simulink subsystem "invertedPendulum"  (R2024a)
settings: Solver=VariableStepAuto  StartTime=0.0  StopTime=10.0  RelTol=1e-3
undefined symbols (not defined in the file): I, L, m, M
settings Model: Creator=Peter  LastModifiedBy=Peter

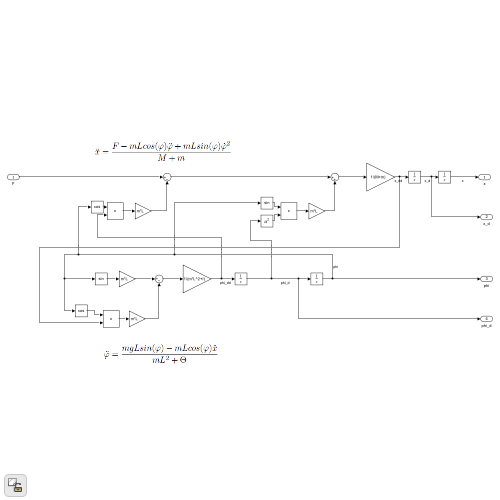
[thumbnail: Simulink's stored preview of the top-level diagram]
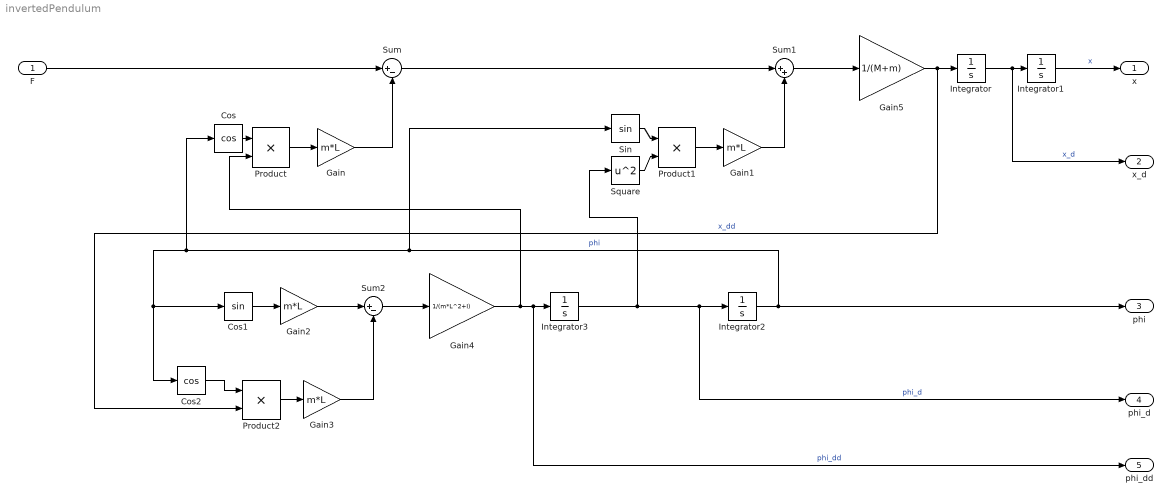
== system invertedPendulum ==
  F : Inport
  Cos : Trigonometry  Operator=cos
  Cos1 : Trigonometry
  Cos2 : Trigonometry  Operator=cos
  Gain{,1..3} (4 alike) : Gain  Gain=m*L
  Gain4 : Gain  Gain=1/(m*L^2+I)
  Gain5 : Gain  Gain=1/(M+m)
  Integrator{,1..3} (4 alike) : Integrator
  Product : Product
  Product1 : Product
  Product2 : Product
  Sin : Trigonometry
  Square : Math  Operator=square
  Sum : Sum  Inputs=|+-
  Sum1 : Sum  Inputs=|++
  Sum2 : Sum  Inputs=|+-
  x : Outport
  x_d : Outport  Port=2
  phi : Outport  Port=3
  phi_d : Outport  Port=4
  phi_dd : Outport  Port=5
  wires:
  Integrator1/1 -> x/1  "x"
  Square/1 -> Product1/2
  Integrator2/1 -> Sin/1, Cos/1, Cos1/1, Cos2/1, phi/1  "phi"
  Sin/1 -> Product1/1
  F/1 -> Sum/1
  Product/1 -> Gain/1
  Gain1/1 -> Sum1/2
  Gain5/1 -> Integrator/1, Product2/2  "x_dd"
  Cos/1 -> Product/1
  Sum/1 -> Sum1/1
  Gain2/1 -> Sum2/1
  Product1/1 -> Gain1/1
  Cos1/1 -> Gain2/1
  Integrator/1 -> Integrator1/1, x_d/1  "x_d"
  Sum2/1 -> Gain4/1
  Integrator3/1 -> Square/1, Integrator2/1, phi_d/1  "phi_d"
  Cos2/1 -> Product2/1
  Gain3/1 -> Sum2/2
  Product2/1 -> Gain3/1
  Gain4/1 -> Integrator3/1, phi_dd/1, Product/2  "phi_dd"
  Gain/1 -> Sum/2
  Sum1/1 -> Gain5/1
